simulink model "FaultCheck"  (R2022b)
settings: Solver=FixedStepAuto  StartTime=0.0  StopTime=10  FixedStep=1  RelTol=1e-3
undefined symbols (not defined in the file): C_Flt_IGBTULowerTempConfirmTh_u16, C_Flt_IGBTULowerTempDiagEn_b, C_Flt_IGBTULowerTempErrCode_u16, C_Flt_IGBTULowerTempPowerCoeff, C_Flt_IGBTULowerTempRecoveryTh_u16, C_Flt_IGBTULowerTempRecTh_s32, C_Flt_IGBTULowerTempTrigTh_s32, C_Flt_IGBTUOverTempConfirmTh_u16, C_Flt_IGBTUOverTempDiagEn_b, C_Flt_IGBTUOverTempErrCode_u16, C_Flt_IGBTUOverTempRecoveryTh_u16, C_Flt_IGBTUOverTempRecTh_s32, C_Flt_IGBTUOverTempTrigTh_s32, C_Flt_IGBTVLowerTempConfirmTh_u16, C_Flt_IGBTVLowerTempDiagEn_b, C_Flt_IGBTVLowerTempErrCode_u16, C_Flt_IGBTVLowerTempPowerCoeff, C_Flt_IGBTVLowerTempRecoveryTh_u16, C_Flt_IGBTVLowerTempRecTh_s32, C_Flt_IGBTVLowerTempTrigTh_s32, C_Flt_IGBTVOverTempConfirmTh_u16, C_Flt_IGBTVOverTempDiagEn_b, C_Flt_IGBTVOverTempErrCode_u16, C_Flt_IGBTVOverTempRecoveryTh_u16, C_Flt_IGBTVOverTempRecTh_s32, C_Flt_IGBTVOverTempTrigTh_s32, C_Flt_IGBTWLowerTempConfirmTh_u16, C_Flt_IGBTWLowerTempDiagEn_b, C_Flt_IGBTWLowerTempErrCode_u16, C_Flt_IGBTWLowerTempPowerCoeff, C_Flt_IGBTWLowerTempRecoveryTh_u16, C_Flt_IGBTWLowerTempRecTh_s32, C_Flt_IGBTWLowerTempTrigTh_s32, C_Flt_IGBTWOverTempConfirmTh_u16, C_Flt_IGBTWOverTempDiagEn_b, C_Flt_IGBTWOverTempErrCode_u16, C_Flt_IGBTWOverTempRecoveryTh_u16, C_Flt_IGBTWOverTempRecTh_s32, C_Flt_IGBTWOverTempTrigTh_s32, C_Flt_IuOCConfirmTh_u16, C_Flt_IuOCDiagEn_b, C_Flt_IuOCErrCode_u16, C_Flt_IuOCNegLimit_s32, C_Flt_IuOCPosLimit_s32, C_Flt_IuOCRecoveryTh_u16, C_Flt_IuZeroDriftDiagEn_b, C_Flt_IuZeroDriftErrCode_u16, C_Flt_IvOCConfirmTh_u16, C_Flt_IvOCDiagEn_b, C_Flt_IvOCErrCode_u16, C_Flt_IvOCNegLimit_s32, C_Flt_IvOCPosLimit_s32, C_Flt_IvOCRecoveryTh_u16, C_Flt_IvZeroDriftDiagEn_b, C_Flt_IvZeroDriftErrCode_u16, C_Flt_IwOCConfirmTh_u16, C_Flt_IwOCDiagEn_b, C_Flt_IwOCErrCode_u16, C_Flt_IwOCNegLimit_s32, C_Flt_IwOCPosLimit_s32 ... (+196)
libraries: YS_UserDefined_Library x21, simulink x5
(part 3 of 11)

== system FaultCheck/FaultDiagnose/UdcOverOneDiag/Diagnose ==
  DiagEnOut : Inport
  Udc : Inport  Port=2
  Parameter : Inport  Port=3
  Disable : Subsystem  TreatAsAtomicUnit=on
  If : If  IfExpression=u1 == 0
  Merge : Merge
  NormalDiag : Subsystem  TreatAsAtomicUnit=on
  UdcOverOneFlgOut : Outport
  wires:
  DiagEnOut/1 -> If/1
  If/1 -> Disable/Action
  If/2 -> NormalDiag/Action
  Udc/1 -> NormalDiag/1(Udc)
  Parameter/1 -> NormalDiag/2(Parameter)
  Disable/1(UdcOverOneFltDeb) -> Merge/1
  NormalDiag/1(UdcOverOneFltDeb) -> Merge/2
  Merge/1 -> UdcOverOneFlgOut/1  "M_Flt_UdcOverOneFlgOut_b"

== system FaultCheck/FaultDiagnose/UdcOverOneDiag/EnableJudgement ==
  SysSelfCheckDownFlg : Inport
  DiagEn : Inport  Port=2
  Constant : Constant  Value=true
  Logical Operator : Logic  AllPortsSameDT=off  OutDataTypeStr=boolean
  Logical Operator1 : Logic  AllPortsSameDT=off  OutDataTypeStr=boolean
  Logical Operator2 : Logic  AllPortsSameDT=off  OutDataTypeStr=boolean
  DiagEnOut : Outport
  wires:
  SysSelfCheckDownFlg/1 -> Logical Operator/2
  DiagEn/1 -> Logical Operator1/2
  Constant/1 -> Logical Operator/1, Logical Operator1/1
  Logical Operator/1 -> Logical Operator2/1
  Logical Operator1/1 -> Logical Operator2/2
  Logical Operator2/1 -> DiagEnOut/1  "M_Flt_UdcOverOneDiagEn_b"

== system FaultCheck/FaultDiagnose/UdcOverOneDiag/FaultLevelDeter ==
  UdcOverOneFlgOut : Inport
  FaultLevel : Inport  Port=2
  If : If  IfExpression=u1 == 0
  Merge : Merge
  Normal : Subsystem  TreatAsAtomicUnit=on
  OverOne : Subsystem  TreatAsAtomicUnit=on
  UdcOverOneFltLevelOut : Outport
  wires:
  UdcOverOneFlgOut/1 -> If/1
  If/1 -> Normal/Action
  If/2 -> OverOne/Action
  Normal/1(UdcOverOneFltLevel) -> Merge/1
  OverOne/1(UdcOverOneFltLevel) -> Merge/2
  Merge/1 -> UdcOverOneFltLevelOut/1  "M_Flt_UdcOverOneFltLevelOut_u8"
  FaultLevel/1 -> OverOne/1(FaultLevel)

== system FaultCheck/FaultDiagnose/UdcOverOneDiag/Parameter ==
  Udc : Inport
  1-D Lookup Table : Lookup_n-D  NumberOfTableDimensions=1  BreakpointsForDimension1=[-5:5]  BreakpointsForDimension1DataTypeStr=Inherit: Inherit from 'Breakpoint data'  IndexSearchMethod=Linear search  Table=tanh([-5:5])  TableDataTypeStr=Inherit: Inherit from 'Table data'  ExtrapMethod=Clip  UseLastTableValue=on  InternalRulePriority=Speed  OutDataTypeStr=single  RndMeth=Simplest
  Bus Creator : BusCreator  Inputs=8
  Constant : Constant  Value=C_Flt_UdcOverOneDiagEn_b
  Constant1 : Constant  Value=C_Flt_UdcOverOneErrCode_u16
  Constant2 : Constant  Value=C_Flt_UdcOverOneConfirmTh_u16
  Constant3 : Constant  Value=C_Flt_UdcOverOneRecoveryTh_u16
  Constant4 : Constant  Value=C_Flt_UdcOverOneTrigTh_s32
  Constant5 : Constant  Value=C_Flt_UdcOverOneRecTh_s32
  Constant6 : Constant  Value=C_Flt_LevelTwo_u8
  Parameter : Outport
  wires:
  Bus Creator/1 -> Parameter/1
  Constant/1 -> Bus Creator/1  "UdcOverOneDiagEn"
  Udc/1 -> 1-D Lookup Table/1
  Constant1/1 -> Bus Creator/2  "UdcOverOneErrCode"
  Constant2/1 -> Bus Creator/5  "UdcOverOneConfirmTh"
  Constant3/1 -> Bus Creator/6  "UdcOverOneRecoveryTh"
  Constant6/1 -> Bus Creator/7  "UdcOverOneFltLevel"
  1-D Lookup Table/1 -> Bus Creator/8  "UdcOverOnePowerCoeff"
  Constant4/1 -> Bus Creator/3  "UdcOverOneTrigTh"
  Constant5/1 -> Bus Creator/4  "UdcOverOneRecTh"

== system FaultCheck/FaultDiagnose/UdcOverOneDiag/PowerReductionCoeffDeter ==
  UdcOverOneFltLevelOut : Inport
  PowerCoeff : Inport  Port=2
  If : If  IfExpression=u1 < 2  ElseIfExpressions=u1 == 2
  If Action Subsystem : Subsystem  TreatAsAtomicUnit=on
  If Action Subsystem1 : Subsystem  TreatAsAtomicUnit=on
  If Action Subsystem2 : Subsystem  TreatAsAtomicUnit=on
  Merge : Merge  Inputs=3
  UdcOverOnePowerCoeffOut : Outport
  wires:
  UdcOverOneFltLevelOut/1 -> If/1
  If/1 -> If Action Subsystem/Action
  If/2 -> If Action Subsystem1/Action
  If/3 -> If Action Subsystem2/Action
  PowerCoeff/1 -> If Action Subsystem1/1(PowerCoeff)
  If Action Subsystem/1(Coeff) -> Merge/1
  If Action Subsystem1/1(Coeff) -> Merge/2
  If Action Subsystem2/1(Coeff) -> Merge/3
  Merge/1 -> UdcOverOnePowerCoeffOut/1  "M_Flt_UdcOverOnePowerCoeffOut_s32"

== system FaultCheck/FaultDiagnose/UdcOverTwoDiag/Diagnose ==
  DiagEnOut : Inport
  Udc : Inport  Port=2
  Parameter : Inport  Port=3
  Disable : Subsystem  TreatAsAtomicUnit=on
  If : If  IfExpression=u1 == 0
  Merge : Merge
  NormalDiag : Subsystem  TreatAsAtomicUnit=on
  UdcOverTwoFlgOut : Outport
  wires:
  DiagEnOut/1 -> If/1
  If/1 -> Disable/Action
  If/2 -> NormalDiag/Action
  Udc/1 -> NormalDiag/1(Udc)
  Parameter/1 -> NormalDiag/2(Parameter)
  Disable/1(UdcOverTwoFltDeb) -> Merge/1
  NormalDiag/1(UdcOverTwoFltDeb) -> Merge/2
  Merge/1 -> UdcOverTwoFlgOut/1  "M_Flt_UdcOverTwoFlgOut_b"

== system FaultCheck/FaultDiagnose/UdcOverTwoDiag/EnableJudgement ==
  SysSelfCheckDownFlg : Inport
  DiagEn : Inport  Port=2
  Constant : Constant  Value=true
  Logical Operator : Logic  AllPortsSameDT=off  OutDataTypeStr=boolean
  Logical Operator1 : Logic  AllPortsSameDT=off  OutDataTypeStr=boolean
  Logical Operator2 : Logic  AllPortsSameDT=off  OutDataTypeStr=boolean
  DiagEnOut : Outport
  wires:
  SysSelfCheckDownFlg/1 -> Logical Operator/2
  DiagEn/1 -> Logical Operator1/2
  Constant/1 -> Logical Operator/1, Logical Operator1/1
  Logical Operator/1 -> Logical Operator2/1
  Logical Operator1/1 -> Logical Operator2/2
  Logical Operator2/1 -> DiagEnOut/1  "M_Flt_UdcOverTwoDiagEn_b"

== system FaultCheck/FaultDiagnose/UdcOverTwoDiag/FaultLevelDeter ==
  UdcOverTwoFlgOut : Inport
  FaultLevel : Inport  Port=2
  If : If  IfExpression=u1 == 0
  Merge : Merge
  Normal : Subsystem  TreatAsAtomicUnit=on
  OverTwo : Subsystem  TreatAsAtomicUnit=on
  UdcOverTwoFltLevelOut : Outport
  wires:
  UdcOverTwoFlgOut/1 -> If/1
  If/1 -> Normal/Action
  If/2 -> OverTwo/Action
  Normal/1(UdcOverTwoFltLevel) -> Merge/1
  OverTwo/1(UdcOverTwoFltLevel) -> Merge/2
  Merge/1 -> UdcOverTwoFltLevelOut/1  "M_Flt_UdcOverTwoFltLevelOut_u8"
  FaultLevel/1 -> OverTwo/1(FaultLevel)

== system FaultCheck/FaultDiagnose/UdcOverTwoDiag/Parameter ==
  Bus Creator : BusCreator  Inputs=7
  Constant : Constant  Value=C_Flt_UdcOverTwoDiagEn_b
  Constant1 : Constant  Value=C_Flt_UdcOverTwoErrCode_u16
  Constant2 : Constant  Value=C_Flt_UdcOverTwoConfirmTh_u16
  Constant3 : Constant  Value=C_Flt_UdcOverTwoRecoveryTh_u16
  Constant4 : Constant  Value=C_Flt_UdcOverTwoTrigTh_s32
  Constant5 : Constant  Value=C_Flt_PowerCoeffZero_s32
  Constant6 : Constant  Value=C_Flt_LevelFive_u8
  Parameter : Outport
  wires:
  Bus Creator/1 -> Parameter/1
  Constant/1 -> Bus Creator/1  "UdcOverTwoDiagEn"
  Constant1/1 -> Bus Creator/2  "UdcOverTwoErrCode"
  Constant2/1 -> Bus Creator/4  "UdcOverTwoConfirmTh"
  Constant3/1 -> Bus Creator/5  "UdcOverTwoRecoveryTh"
  Constant6/1 -> Bus Creator/6  "UdcOverTwoFltLevel"
  Constant5/1 -> Bus Creator/7  "UdcOverTwoPowerCoeff"
  Constant4/1 -> Bus Creator/3  "UdcOverTwoTrigTh"

== system FaultCheck/FaultDiagnose/UdcOverTwoDiag/PowerReductionCoeffDeter ==
  UdcOverTwoFltLevelOut : Inport
  PowerCoeff : Inport  Port=2
  If : If  IfExpression=u1 < 2  ElseIfExpressions=u1 == 2
  If Action Subsystem : Subsystem  TreatAsAtomicUnit=on
  If Action Subsystem1 : Subsystem  TreatAsAtomicUnit=on
  If Action Subsystem2 : Subsystem  TreatAsAtomicUnit=on
  Merge : Merge  Inputs=3
  UdcOverTwoPowerCoeffOut : Outport
  wires:
  UdcOverTwoFltLevelOut/1 -> If/1
  If/1 -> If Action Subsystem/Action
  If/2 -> If Action Subsystem1/Action
  If/3 -> If Action Subsystem2/Action
  PowerCoeff/1 -> If Action Subsystem1/1(PowerCoeff)
  If Action Subsystem/1(Coeff) -> Merge/1
  If Action Subsystem1/1(Coeff) -> Merge/2
  If Action Subsystem2/1(Coeff) -> Merge/3
  Merge/1 -> UdcOverTwoPowerCoeffOut/1  "M_Flt_UdcOverTwoPowerCoeffOut_s32"

== system FaultCheck/FltCheck/Determination/Detection Criteria ==
  FltSrc : Inport
  FltTh : Inport  Port=2
  Condition : Inport  Port=3
  Determination : Subsystem
  Equal : Subsystem
  Lower : Subsystem
  NotEqual : Subsystem
  Overflow : Subsystem
  Fail : Outport
  wires:
  FltTh/1 -> NotEqual/2(FltTh), Lower/2(FltTh), Overflow/2(FltTh), Equal/2(FltTh)
  FltSrc/1 -> NotEqual/1(FltSrc), Lower/1(FltSrc), Overflow/1(FltSrc), Equal/1(FltSrc)
  Equal/1(EQ) -> Determination/2(EQ)
  Overflow/1(GT) -> Determination/3(GT)
  Lower/1(LT) -> Determination/4(LT)
  NotEqual/1(NEQ) -> Determination/5(NEQ)
  Condition/1 -> Determination/1(Condition)
  Determination/1(Fail) -> Fail/1

== system FaultCheck/FltCheck/Determination/Hysteresis ==
  Fail : Inport
  ConfirmTh : Inport  Port=2
  ClearTh : Inport  Port=3
  FastRecover_one : Inport  Port=4
  Hysteresis_Chart : Stateflow chart  TreatAsAtomicUnit=on
  Out : Outport
  wires:
  Fail/1 -> Hysteresis_Chart/1(Fail)
  ClearTh/1 -> Hysteresis_Chart/2(ClearTh)
  ConfirmTh/1 -> Hysteresis_Chart/3(ConfirmTh)
  FastRecover_one/1 -> Hysteresis_Chart/4(FastRecover_one)
  Hysteresis_Chart/1(Out) -> Out/1

== system FaultCheck/FaultDiag_HighTask_100us/FltDetn/CurrentSensorDetn/Enable ==
  Sys_SelfChkFishFlg : Inport
  Constant : Constant  Value=FLT_ON
  Constant1 : Constant  Value=FLT_ON
  Constant2 : Constant  Value=FLT_OFF
  Relational Operator : RelationalOperator  Operator===  OutDataTypeStr=boolean  RndMeth=Simplest  InputSameDT=off
  Switch : Switch  Criteria=u2 > Threshold  SaturateOnIntegerOverflow=off  InputSameDT=off
  Enable : Outport
  wires:
  Switch/1 -> Enable/1
  Constant2/1 -> Switch/3
  Constant1/1 -> Switch/1
  Relational Operator/1 -> Switch/2
  Constant/1 -> Relational Operator/2
  Sys_SelfChkFishFlg/1 -> Relational Operator/1

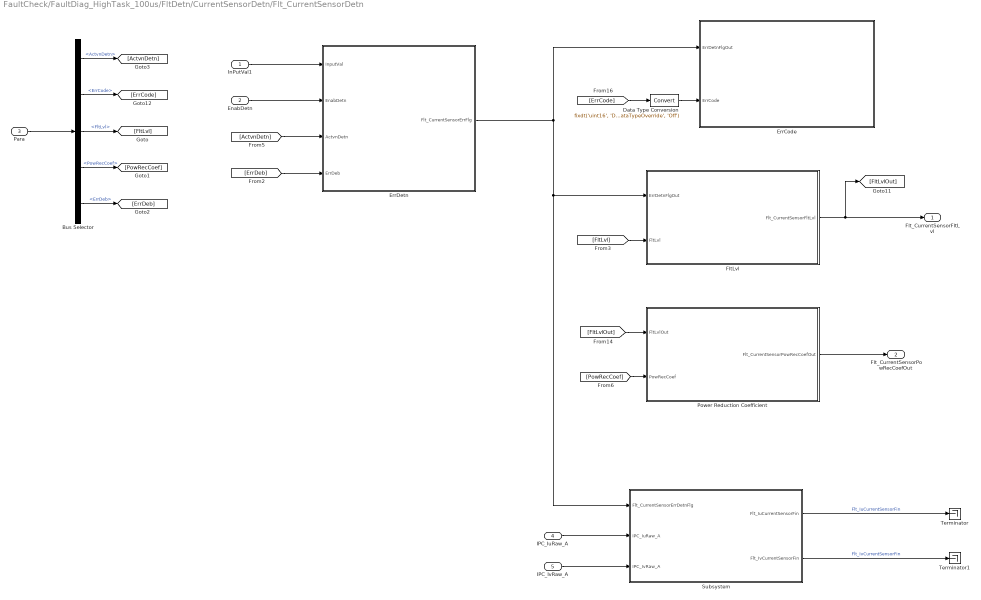
== system FaultCheck/FaultDiag_HighTask_100us/FltDetn/CurrentSensorDetn/Flt_CurrentSensorDetn ==
  InPutVal1 : Inport
  EnabDetn : Inport  Port=2
  Para : Inport  Port=3
  IPC_IuRaw_A : Inport  Port=4
  IPC_IvRaw_A : Inport  Port=5
  Bus Selector : BusSelector  OutputSignals=ActvnDetn,ErrCode,FltLvl,PowRecCoef,ErrDeb
  Data Type Conversion : DataTypeConversion  OutDataTypeStr=fixdt('uint16', 'DataTypeOverride', 'Off')  SaturateOnIntegerOverflow=off  RndMeth=Floor
  ErrCode : Subsystem
  ErrDetn : Subsystem
  FltLvl : Subsystem
  Power Reduction Coefficient : Subsystem
  Subsystem : Subsystem
  Terminator : Terminator
  Terminator1 : Terminator
  Flt_CurrentSensorFltLvl : Outport
  Flt_CurrentSensorPowRecCoefOut : Outport  Port=2
  wires:
  Subsystem/2(Flt_IvCurrentSensorFin) -> Terminator1/1  "Flt_IvCurrentSensorFin"
  IPC_IvRaw_A/1 -> Subsystem/3(IPC_IvRaw_A)
  IPC_IuRaw_A/1 -> Subsystem/2(IPC_IuRaw_A)
  Subsystem/1(Flt_IuCurrentSensorFin) -> Terminator/1  "Flt_IuCurrentSensorFin"
  ErrDetn/1(Flt_CurrentSensorErrFlg) -> Subsystem/1(Flt_CurrentSensorErrDetnFlg), FltLvl/1(ErrDetnFlgOut), ErrCode/1(ErrDetnFlgOut)
  Bus Selector/5 -> [ErrDeb]  "<ErrDeb>"
  InPutVal1/1 -> ErrDetn/1(InputVal)
  [ActvnDetn] -> ErrDetn/3(ActvnDetn)
  EnabDetn/1 -> ErrDetn/2(EnabDetn)
  [ErrDeb] -> ErrDetn/4(ErrDeb)
  Bus Selector/4 -> [PowRecCoef]  "<PowRecCoef>"
  Bus Selector/3 -> [FltLvl]  "<FltLvl>"
  Bus Selector/2 -> [ErrCode]  "<ErrCode>"
  Bus Selector/1 -> [ActvnDetn]  "<ActvnDetn>"
  Para/1 -> Bus Selector/1
  [ErrCode] -> Data Type Conversion/1
  FltLvl/1(Flt_CurrentSensorFltLvl) -> [FltLvlOut], Flt_CurrentSensorFltLvl/1
  [FltLvl] -> FltLvl/2(FltLvl)
  [FltLvlOut] -> Power Reduction Coefficient/1(FltLvlOut)
  [PowRecCoef] -> Power Reduction Coefficient/2(PowRecCoef)
  Power Reduction Coefficient/1(Flt_CurrentSensorPowRecCoefOut) -> Flt_CurrentSensorPowRecCoefOut/1
  Data Type Conversion/1 -> ErrCode/2(ErrCode)

== system FaultCheck/FaultDiag_HighTask_100us/FltDetn/CurrentSensorDetn/Parameter ==
  Bus Creator : BusCreator  Inputs=5
  Constant2 : Constant  Value=FLT_COEF_ZERO
  Constant3 : Constant  Value=Flt_CurrentSensor_ErrCode
  Constant4 : Constant  Value=FLTLVL_FOUR
  Constant5 : Constant  Value=Flt_CurrentSensor_ActvnDetn
  Constant8 : Constant  Value=Flt_CurrentSensor_ErrDeb
  Para : Outport
  wires:
  Constant8/1 -> Bus Creator/1  "ErrDeb"
  Constant2/1 -> Bus Creator/5  "PowRecCoef"
  Constant3/1 -> Bus Creator/3  "ErrCode"
  Constant5/1 -> Bus Creator/2  "ActvnDetn"
  Constant4/1 -> Bus Creator/4  "FltLvl"
  Bus Creator/1 -> Para/1

== system FaultCheck/FaultDiag_HighTask_100us/FltDetn/CurrentZeroDrfDetn/CurrZeroDrfDetn ==
  InPutVal : Inport
  EnabDetn : Inport  Port=2
  Para : Inport  Port=3
  Bus Selector : BusSelector  OutputSignals=ActvnDetn,ErrCode,FltLvl,PowRecCoef
  ErrCode1 : Subsystem
  ErrDetn : Subsystem
  FltLvl : Subsystem
  Power Reduction Coefficient : Subsystem
  Flt_CurrZeroDrfFltLvl : Outport
  Flt_CurrZeroDrfPowRecCoefOut : Outport  Port=2
  wires:
  ErrDetn/1(Flt_CurrZeroDrfErrFlg) -> FltLvl/1(ErrDetnFlgOut), ErrCode1/1(ErrDetnFlgOut)
  InPutVal/1 -> ErrDetn/1(InputVal)
  [ActvnDetn] -> ErrDetn/3(ActvnDetn)
  EnabDetn/1 -> ErrDetn/2(EnabDetn)
  Bus Selector/4 -> [PowRecCoef]  "<PowRecCoef>"
  Bus Selector/3 -> [FltLvl]  "<FltLvl>"
  Bus Selector/2 -> [ErrCode]  "<ErrCode>"
  Bus Selector/1 -> [ActvnDetn]  "<ActvnDetn>"
  Para/1 -> Bus Selector/1
  [ErrCode] -> ErrCode1/2(ErrCode)
  FltLvl/1(Flt_CurrZeroDrfFltLvl) -> [FltLvlOut], Flt_CurrZeroDrfFltLvl/1
  [FltLvl] -> FltLvl/2(FltLvl)
  [FltLvlOut] -> Power Reduction Coefficient/1(FltLvlOut)
  [PowRecCoef] -> Power Reduction Coefficient/2(PowRecCoef)
  Power Reduction Coefficient/1(Flt_CurrZeroDrfPowRecCoefOut) -> Flt_CurrZeroDrfPowRecCoefOut/1

== system FaultCheck/FaultDiag_HighTask_100us/FltDetn/CurrentZeroDrfDetn/Enable ==
  Constant : Constant  Value=FLT_ON
  Enable : Outport
  wires:
  Constant/1 -> Enable/1

== system FaultCheck/FaultDiag_HighTask_100us/FltDetn/CurrentZeroDrfDetn/Parameter ==
  Bus Creator : BusCreator  Inputs=4
  Constant2 : Constant  Value=FLT_COEF_ZERO
  Constant3 : Constant  Value=Flt_CurrZeroDrf_ErrCode
  Constant4 : Constant  Value=FLTLVL_FIVE
  Constant5 : Constant  Value=Flt_CurrZeroDrf_ActvnErrDetn
  Para : Outport
  wires:
  Constant2/1 -> Bus Creator/4  "PowRecCoef"
  Constant3/1 -> Bus Creator/2  "ErrCode"
  Constant5/1 -> Bus Creator/1  "ActvnDetn"
  Constant4/1 -> Bus Creator/3  "FltLvl"
  Bus Creator/1 -> Para/1

== system FaultCheck/FaultDiag_HighTask_100us/FltDetn/DriveUdcDetn/DriveUdcDetn ==
  InPutVal1 : Inport
  EnabDetn : Inport  Port=2
  Para : Inport  Port=3
  Bus Selector : BusSelector  OutputSignals=ActvnDetn,ErrCode,FltLvl,PowRecCoef,ErrDeb
  ErrCode : Subsystem
  ErrDetn : Subsystem
  FltLvl : Subsystem
  Power Reduction Coefficient : Subsystem
  Flt_DriveUdcFltLvl : Outport
  Flt_DriveUdcPowRecCoefOut : Outport  Port=2
  wires:
  Power Reduction Coefficient/1(Flt_DriveUdcPowRecCoefOut) -> Flt_DriveUdcPowRecCoefOut/1
  [PowRecCoef] -> Power Reduction Coefficient/2(PowRecCoef)
  [FltLvlOut] -> Power Reduction Coefficient/1(FltLvlOut)
  [FltLvl] -> FltLvl/2(FltLvl)
  FltLvl/1(Flt_DriveUdcFltLvl) -> Flt_DriveUdcFltLvl/1, [FltLvlOut]
  [ErrCode] -> ErrCode/2(ErrCode)
  Para/1 -> Bus Selector/1
  Bus Selector/1 -> [ActvnDetn]  "<ActvnDetn>"
  Bus Selector/2 -> [ErrCode]  "<ErrCode>"
  Bus Selector/3 -> [FltLvl]  "<FltLvl>"
  Bus Selector/4 -> [PowRecCoef]  "<PowRecCoef>"
  [ErrDeb] -> ErrDetn/4(ErrDeb)
  EnabDetn/1 -> ErrDetn/2(EnabDetn)
  [ActvnDetn] -> ErrDetn/3(ActvnDetn)
  InPutVal1/1 -> ErrDetn/1(InputVal)
  ErrDetn/1(Flt_DriveUdcErrFlg) -> ErrCode/1(ErrDetnFlgOut), FltLvl/1(ErrDetnFlgOut)
  Bus Selector/5 -> [ErrDeb]  "<ErrDeb>"

== system FaultCheck/FaultDiag_HighTask_100us/FltDetn/DriveUdcDetn/Enable ==
  Sys_SelfChkFishFlg : Inport
  Constant : Constant  Value=FLT_ON
  Constant1 : Constant  Value=FLT_ON
  Constant2 : Constant  Value=FLT_OFF
  Relational Operator : RelationalOperator  Operator===  OutDataTypeStr=boolean  RndMeth=Simplest  InputSameDT=off
  Switch : Switch  Criteria=u2 > Threshold  SaturateOnIntegerOverflow=off  InputSameDT=off
  Enable : Outport
  wires:
  Sys_SelfChkFishFlg/1 -> Relational Operator/1
  Constant/1 -> Relational Operator/2
  Relational Operator/1 -> Switch/2
  Constant1/1 -> Switch/1
  Constant2/1 -> Switch/3
  Switch/1 -> Enable/1

== system FaultCheck/FaultDiag_HighTask_100us/FltDetn/DriveUdcDetn/Parameter ==
  Bus Creator : BusCreator  Inputs=5
  Constant2 : Constant  Value=FLT_COEF_ZERO
  Constant3 : Constant  Value=Flt_DriveUdc_ErrCode
  Constant4 : Constant  Value=FLTLVL_FOUR
  Constant5 : Constant  Value=Flt_DriveUdc_ActvnDetn
  Constant8 : Constant  Value=Flt_DriveUdc_ErrDeb
  Para : Outport
  wires:
  Bus Creator/1 -> Para/1
  Constant4/1 -> Bus Creator/4  "FltLvl"
  Constant5/1 -> Bus Creator/2  "ActvnDetn"
  Constant3/1 -> Bus Creator/3  "ErrCode"
  Constant2/1 -> Bus Creator/5  "PowRecCoef"
  Constant8/1 -> Bus Creator/1  "ErrDeb"

== system FaultCheck/FaultDiag_HighTask_100us/FltDetn/Drive_H_Detn/Drive_H_Detn ==
  InPutVal1 : Inport
  EnabDetn : Inport  Port=2
  Para : Inport  Port=3
  Bus Selector : BusSelector  OutputSignals=ActvnDetn,ErrCode,FltLvl,PowRecCoef,ErrDeb
  ErrCode : Subsystem
  ErrDetn : Subsystem
  FltLvl : Subsystem
  Power Reduction Coefficient : Subsystem
  Flt_Drive_H_FltLvl : Outport
  Flt_Drive_H_PowRecCoefOut : Outport  Port=2
  wires:
  Power Reduction Coefficient/1(Flt_Drive_H_PowRecCoefOut) -> Flt_Drive_H_PowRecCoefOut/1
  [PowRecCoef] -> Power Reduction Coefficient/2(PowRecCoef)
  [FltLvlOut] -> Power Reduction Coefficient/1(FltLvlOut)
  [FltLvl] -> FltLvl/2(FltLvl)
  FltLvl/1(Flt_Drive_H_FltLvl) -> Flt_Drive_H_FltLvl/1, [FltLvlOut]
  [ErrCode] -> ErrCode/2(ErrCode)
  Para/1 -> Bus Selector/1
  Bus Selector/1 -> [ActvnDetn]  "<ActvnDetn>"
  Bus Selector/2 -> [ErrCode]  "<ErrCode>"
  Bus Selector/3 -> [FltLvl]  "<FltLvl>"
  Bus Selector/4 -> [PowRecCoef]  "<PowRecCoef>"
  [ErrDeb] -> ErrDetn/4(ErrDeb)
  EnabDetn/1 -> ErrDetn/2(EnabDetn)
  [ActvnDetn] -> ErrDetn/3(ActvnDetn)
  InPutVal1/1 -> ErrDetn/1(InputVal)
  ErrDetn/1(Flt_Drive_H_ErrFlg) -> ErrCode/1(ErrDetnFlgOut), FltLvl/1(ErrDetnFlgOut)
  Bus Selector/5 -> [ErrDeb]  "<ErrDeb>"

== system FaultCheck/FaultDiag_HighTask_100us/FltDetn/Drive_H_Detn/Enable ==
  Sys_SelfChkFishFlg : Inport
  Constant : Constant  Value=FLT_ON
  Constant1 : Constant  Value=FLT_ON
  Constant2 : Constant  Value=FLT_OFF
  Relational Operator : RelationalOperator  Operator===  OutDataTypeStr=boolean  RndMeth=Simplest  InputSameDT=off
  Switch : Switch  Criteria=u2 > Threshold  SaturateOnIntegerOverflow=off  InputSameDT=off
  Enable : Outport
  wires:
  Sys_SelfChkFishFlg/1 -> Relational Operator/1
  Constant/1 -> Relational Operator/2
  Relational Operator/1 -> Switch/2
  Constant1/1 -> Switch/1
  Constant2/1 -> Switch/3
  Switch/1 -> Enable/1

== system FaultCheck/FaultDiag_HighTask_100us/FltDetn/Drive_H_Detn/Parameter ==
  Bus Creator : BusCreator  Inputs=5
  Constant2 : Constant  Value=FLT_COEF_ZERO
  Constant3 : Constant  Value=Flt_Drive_H_ErrCode
  Constant4 : Constant  Value=FLTLVL_FOUR
  Constant5 : Constant  Value=Flt_Drive_H_ActvnDetn
  Constant8 : Constant  Value=Flt_Drive_H_ErrDeb
  Para : Outport
  wires:
  Bus Creator/1 -> Para/1
  Constant4/1 -> Bus Creator/4  "FltLvl"
  Constant5/1 -> Bus Creator/2  "ActvnDetn"
  Constant3/1 -> Bus Creator/3  "ErrCode"
  Constant2/1 -> Bus Creator/5  "PowRecCoef"
  Constant8/1 -> Bus Creator/1  "ErrDeb"

== system FaultCheck/FaultDiag_HighTask_100us/FltDetn/Drive_L_Detn/Drive_L_Detn ==
  InPutVal1 : Inport
  EnabDetn : Inport  Port=2
  Para : Inport  Port=3
  Bus Selector : BusSelector  OutputSignals=ActvnDetn,ErrCode,FltLvl,PowRecCoef,ErrDeb
  ErrCode : Subsystem
  ErrDetn : Subsystem
  FltLvl : Subsystem
  Power Reduction Coefficient : Subsystem
  Flt_Drive_L_FltLvl : Outport
  Flt_Drive_L_PowRecCoefOut : Outport  Port=2
  wires:
  Power Reduction Coefficient/1(Flt_Drive_L_PowRecCoefOut) -> Flt_Drive_L_PowRecCoefOut/1
  [PowRecCoef] -> Power Reduction Coefficient/2(PowRecCoef)
  [FltLvlOut] -> Power Reduction Coefficient/1(FltLvlOut)
  [FltLvl] -> FltLvl/2(FltLvl)
  FltLvl/1(Flt_Drive_L_FltLvl) -> Flt_Drive_L_FltLvl/1, [FltLvlOut]
  [ErrCode] -> ErrCode/2(ErrCode)
  Para/1 -> Bus Selector/1
  Bus Selector/1 -> [ActvnDetn]  "<ActvnDetn>"
  Bus Selector/2 -> [ErrCode]  "<ErrCode>"
  Bus Selector/3 -> [FltLvl]  "<FltLvl>"
  Bus Selector/4 -> [PowRecCoef]  "<PowRecCoef>"
  [ErrDeb] -> ErrDetn/4(ErrDeb)
  EnabDetn/1 -> ErrDetn/2(EnabDetn)
  [ActvnDetn] -> ErrDetn/3(ActvnDetn)
  InPutVal1/1 -> ErrDetn/1(InputVal)
  ErrDetn/1(Flt_Drive_L_ErrFlg) -> ErrCode/1(ErrDetnFlgOut), FltLvl/1(ErrDetnFlgOut)
  Bus Selector/5 -> [ErrDeb]  "<ErrDeb>"

== system FaultCheck/FaultDiag_HighTask_100us/FltDetn/Drive_L_Detn/Enable ==
  Sys_SelfChkFishFlg : Inport
  Constant : Constant  Value=FLT_ON
  Constant1 : Constant  Value=FLT_ON
  Constant2 : Constant  Value=FLT_OFF
  Relational Operator : RelationalOperator  Operator===  OutDataTypeStr=boolean  RndMeth=Simplest  InputSameDT=off
  Switch : Switch  Criteria=u2 > Threshold  SaturateOnIntegerOverflow=off  InputSameDT=off
  Enable : Outport
  wires:
  Sys_SelfChkFishFlg/1 -> Relational Operator/1
  Constant/1 -> Relational Operator/2
  Relational Operator/1 -> Switch/2
  Constant1/1 -> Switch/1
  Constant2/1 -> Switch/3
  Switch/1 -> Enable/1

== system FaultCheck/FaultDiag_HighTask_100us/FltDetn/Drive_L_Detn/Parameter ==
  Bus Creator : BusCreator  Inputs=5
  Constant2 : Constant  Value=FLT_COEF_ZERO
  Constant3 : Constant  Value=Flt_Drive_L_ErrCode
  Constant4 : Constant  Value=FLTLVL_FOUR
  Constant5 : Constant  Value=Flt_Drive_L_ActvnDetn
  Constant8 : Constant  Value=Flt_Drive_L_ErrDeb
  Para : Outport
  wires:
  Bus Creator/1 -> Para/1
  Constant4/1 -> Bus Creator/4  "FltLvl"
  Constant5/1 -> Bus Creator/2  "ActvnDetn"
  Constant3/1 -> Bus Creator/3  "ErrCode"
  Constant2/1 -> Bus Creator/5  "PowRecCoef"
  Constant8/1 -> Bus Creator/1  "ErrDeb"

== system FaultCheck/FaultDiag_HighTask_100us/FltDetn/HWOverCurrDetn/Enable ==
  Sys_SelfChkFishFlg : Inport
  Constant : Constant  Value=FLT_ON
  Constant1 : Constant  Value=FLT_ON
  Constant2 : Constant  Value=FLT_OFF
  Relational Operator : RelationalOperator  Operator===  OutDataTypeStr=boolean  RndMeth=Simplest  InputSameDT=off
  Switch : Switch  Criteria=u2 > Threshold  SaturateOnIntegerOverflow=off  InputSameDT=off
  Enable : Outport
  wires:
  Sys_SelfChkFishFlg/1 -> Relational Operator/1
  Constant/1 -> Relational Operator/2
  Relational Operator/1 -> Switch/2
  Constant1/1 -> Switch/1
  Constant2/1 -> Switch/3
  Switch/1 -> Enable/1

== system FaultCheck/FaultDiag_HighTask_100us/FltDetn/HWOverCurrDetn/HWOverCurrDetn ==
  InPutVal1 : Inport
  EnabDetn : Inport  Port=2
  Para : Inport  Port=3
  Bus Selector : BusSelector  OutputSignals=ActvnDetn,ErrCode,FltLvl,PowRecCoef,ErrDeb
  ErrCode : Subsystem
  ErrDetn : Subsystem
  FltLvl : Subsystem
  Power Reduction Coefficient : Subsystem
  Flt_HWOverCurrFltLvl : Outport
  Flt_HWOverCurrPowRecCoefOut : Outport  Port=2
  wires:
  Power Reduction Coefficient/1(Flt_HWOverCurrPowRecCoefOut) -> Flt_HWOverCurrPowRecCoefOut/1
  [PowRecCoef] -> Power Reduction Coefficient/2(PowRecCoef)
  [FltLvlOut] -> Power Reduction Coefficient/1(FltLvlOut)
  [FltLvl] -> FltLvl/2(FltLvl)
  FltLvl/1(Flt_HWOverCurrFltLvl) -> Flt_HWOverCurrFltLvl/1, [FltLvlOut]
  [ErrCode] -> ErrCode/2(ErrCode)
  Para/1 -> Bus Selector/1
  Bus Selector/1 -> [ActvnDetn]  "<ActvnDetn>"
  Bus Selector/2 -> [ErrCode]  "<ErrCode>"
  Bus Selector/3 -> [FltLvl]  "<FltLvl>"
  Bus Selector/4 -> [PowRecCoef]  "<PowRecCoef>"
  [ErrDeb] -> ErrDetn/4(ErrDeb)
  EnabDetn/1 -> ErrDetn/2(EnabDetn)
  [ActvnDetn] -> ErrDetn/3(ActvnDetn)
  InPutVal1/1 -> ErrDetn/1(InputVal)
  ErrDetn/1(Flt_HWOverCurrErrFlg) -> ErrCode/1(ErrDetnFlgOut), FltLvl/1(ErrDetnFlgOut)
  Bus Selector/5 -> [ErrDeb]  "<ErrDeb>"

== system FaultCheck/FaultDiag_HighTask_100us/FltDetn/HWOverCurrDetn/Parameter ==
  Bus Creator : BusCreator  Inputs=5
  Constant2 : Constant  Value=FLT_COEF_ZERO
  Constant3 : Constant  Value=Flt_HWOverCurr_ErrCode
  Constant4 : Constant  Value=FLTLVL_FOUR
  Constant5 : Constant  Value=Flt_HWOverCurr_ActvnDetn
  Constant8 : Constant  Value=Flt_HWOverCurr_ErrDeb
  Para : Outport
  wires:
  Bus Creator/1 -> Para/1
  Constant4/1 -> Bus Creator/4  "FltLvl"
  Constant5/1 -> Bus Creator/2  "ActvnDetn"
  Constant3/1 -> Bus Creator/3  "ErrCode"
  Constant2/1 -> Bus Creator/5  "PowRecCoef"
  Constant8/1 -> Bus Creator/1  "ErrDeb"

== system FaultCheck/FaultDiag_HighTask_100us/FltDetn/HWOverUdcDetn/Enable ==
  Sys_SelfChkFishFlg : Inport
  Constant : Constant  Value=FLT_ON
  Constant1 : Constant  Value=FLT_ON
  Constant2 : Constant  Value=FLT_OFF
  Relational Operator : RelationalOperator  Operator===  OutDataTypeStr=boolean  RndMeth=Simplest  InputSameDT=off
  Switch : Switch  Criteria=u2 > Threshold  SaturateOnIntegerOverflow=off  InputSameDT=off
  Enable : Outport
  wires:
  Sys_SelfChkFishFlg/1 -> Relational Operator/1
  Constant/1 -> Relational Operator/2
  Relational Operator/1 -> Switch/2
  Constant1/1 -> Switch/1
  Constant2/1 -> Switch/3
  Switch/1 -> Enable/1

== system FaultCheck/FaultDiag_HighTask_100us/FltDetn/HWOverUdcDetn/HWOverCurrDetn ==
  InPutVal1 : Inport
  EnabDetn : Inport  Port=2
  Para : Inport  Port=3
  Bus Selector : BusSelector  OutputSignals=ActvnDetn,ErrCode,FltLvl,PowRecCoef,ErrDeb
  ErrCode : Subsystem
  ErrDetn : Subsystem
  FltLvl : Subsystem
  Power Reduction Coefficient : Subsystem
  Flt_HWOverUdcFltLvl : Outport
  Flt_HWOverUdcPowRecCoefOut : Outport  Port=2
  wires:
  Power Reduction Coefficient/1(Flt_HWOverUdcPowRecCoefOut) -> Flt_HWOverUdcPowRecCoefOut/1
  [PowRecCoef] -> Power Reduction Coefficient/2(PowRecCoef)
  [FltLvlOut] -> Power Reduction Coefficient/1(FltLvlOut)
  [FltLvl] -> FltLvl/2(FltLvl)
  FltLvl/1(Flt_HWOverUdcFltLvl) -> Flt_HWOverUdcFltLvl/1, [FltLvlOut]
  [ErrCode] -> ErrCode/2(ErrCode)
  Para/1 -> Bus Selector/1
  Bus Selector/1 -> [ActvnDetn]  "<ActvnDetn>"
  Bus Selector/2 -> [ErrCode]  "<ErrCode>"
  Bus Selector/3 -> [FltLvl]  "<FltLvl>"
  Bus Selector/4 -> [PowRecCoef]  "<PowRecCoef>"
  [ErrDeb] -> ErrDetn/4(ErrDeb)
  EnabDetn/1 -> ErrDetn/2(EnabDetn)
  [ActvnDetn] -> ErrDetn/3(ActvnDetn)
  InPutVal1/1 -> ErrDetn/1(InputVal)
  ErrDetn/1(Flt_HWOverUdcErrFlg) -> ErrCode/1(ErrDetnFlgOut), FltLvl/1(ErrDetnFlgOut)
  Bus Selector/5 -> [ErrDeb]  "<ErrDeb>"

== system FaultCheck/FaultDiag_HighTask_100us/FltDetn/HWOverUdcDetn/Parameter ==
  Bus Creator : BusCreator  Inputs=5
  Constant2 : Constant  Value=FLT_COEF_ZERO
  Constant3 : Constant  Value=Flt_HWOverUdc_ErrCode
  Constant4 : Constant  Value=FLTLVL_FIVE
  Constant5 : Constant  Value=Flt_HWOverUdc_ActvnDetn
  Constant8 : Constant  Value=Flt_HWOverUdc_ErrDeb
  Para : Outport
  wires:
  Bus Creator/1 -> Para/1
  Constant4/1 -> Bus Creator/4  "FltLvl"
  Constant5/1 -> Bus Creator/2  "ActvnDetn"
  Constant3/1 -> Bus Creator/3  "ErrCode"
  Constant2/1 -> Bus Creator/5  "PowRecCoef"
  Constant8/1 -> Bus Creator/1  "ErrDeb"

== system FaultCheck/FaultDiag_HighTask_100us/FltDetn/OverCurrDetn/Enable ==
  Sys_SelfChkFishFlg : Inport
  Constant : Constant  Value=FLT_ON
  Constant1 : Constant  Value=FLT_ON
  Constant2 : Constant  Value=FLT_OFF
  Relational Operator : RelationalOperator  Operator===  OutDataTypeStr=boolean  RndMeth=Simplest  InputSameDT=off
  Switch : Switch  Criteria=u2 > Threshold  SaturateOnIntegerOverflow=off  InputSameDT=off
  Enable : Outport
  wires:
  Sys_SelfChkFishFlg/1 -> Relational Operator/1
  Constant/1 -> Relational Operator/2
  Relational Operator/1 -> Switch/2
  Constant1/1 -> Switch/1
  Constant2/1 -> Switch/3
  Switch/1 -> Enable/1

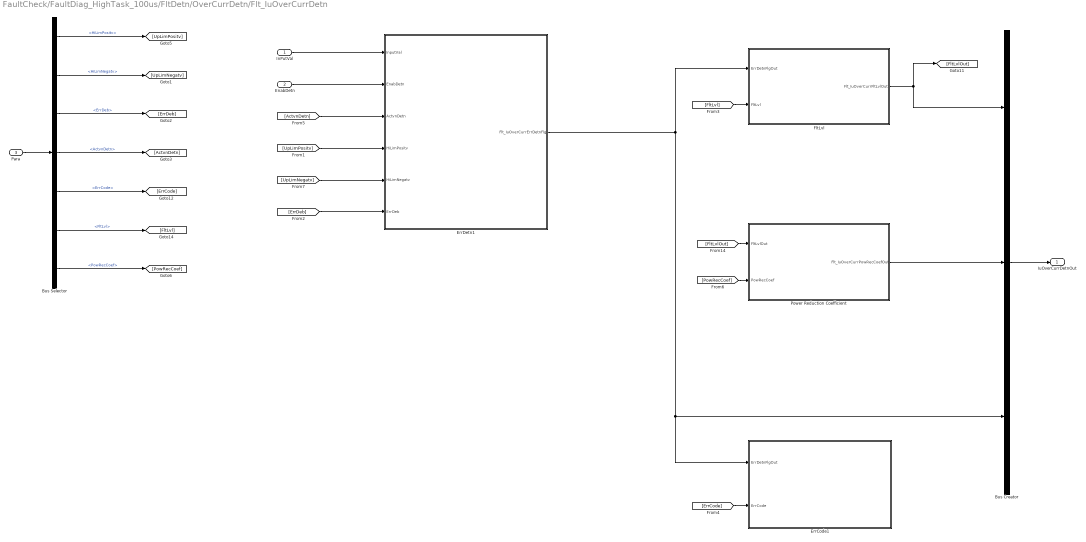
== system FaultCheck/FaultDiag_HighTask_100us/FltDetn/OverCurrDetn/Flt_IuOverCurrDetn ==
  InPutVal : Inport
  EnabDetn : Inport  Port=2
  Para : Inport  Port=3
  Bus Creator : BusCreator  Inputs=3
  Bus Selector : BusSelector  OutputSignals=HiLimPositv,HiLimNegatv,ErrDeb,ActvnDetn,ErrCode,FltLvl,PowRecCoef
  ErrCode1 : Subsystem
  ErrDetn1 : Subsystem
  FltLvl : Subsystem
  Power Reduction Coefficient : Subsystem
  IuOverCurrDetnOut : Outport
  wires:
  Para/1 -> Bus Selector/1
  Bus Selector/2 -> [UpLimNegatv]  "<HiLimNegatv>"
  Bus Selector/3 -> [ErrDeb]  "<ErrDeb>"
  ErrDetn1/1(Flt_IuOverCurrErrDetnFlg) -> Bus Creator/3, ErrCode1/1(ErrDetnFlgOut), FltLvl/1(ErrDetnFlgOut)
  FltLvl/1(Flt_IuOverCurrFltLvlOut) -> Bus Creator/1, [FltLvlOut]
  Bus Selector/5 -> [ErrCode]  "<ErrCode>"
  Bus Selector/6 -> [FltLvl]  "<FltLvl>"
  [FltLvl] -> FltLvl/2(FltLvl)
  [PowRecCoef] -> Power Reduction Coefficient/2(PowRecCoef)
  [FltLvlOut] -> Power Reduction Coefficient/1(FltLvlOut)
  [ErrDeb] -> ErrDetn1/6(ErrDeb)
  [ErrCode] -> ErrCode1/2(ErrCode)
  Power Reduction Coefficient/1(Flt_IuOverCurrPowRecCoefOut) -> Bus Creator/2
  Bus Creator/1 -> IuOverCurrDetnOut/1
  [UpLimNegatv] -> ErrDetn1/5(HiLimNegatv)
  InPutVal/1 -> ErrDetn1/1(InputVal)
  [ActvnDetn] -> ErrDetn1/3(ActvnDetn)
  EnabDetn/1 -> ErrDetn1/2(EnabDetn)
  [UpLimPositv] -> ErrDetn1/4(HiLimPositv)
  Bus Selector/1 -> [UpLimPositv]  "<HiLimPositv>"
  Bus Selector/4 -> [ActvnDetn]  "<ActvnDetn>"
  Bus Selector/7 -> [PowRecCoef]  "<PowRecCoef>"

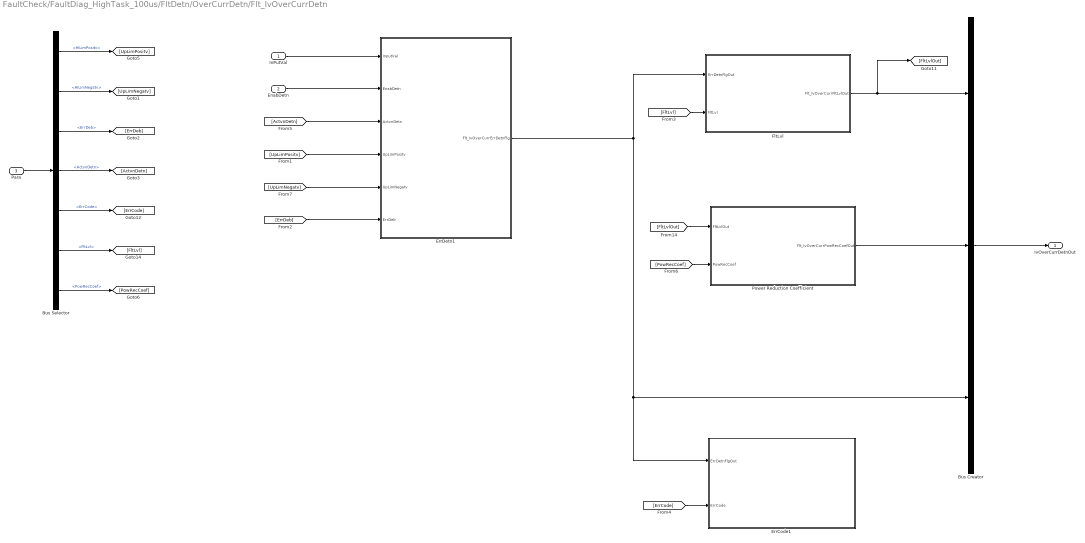
== system FaultCheck/FaultDiag_HighTask_100us/FltDetn/OverCurrDetn/Flt_IvOverCurrDetn ==
  InPutVal : Inport
  EnabDetn : Inport  Port=2
  Para : Inport  Port=3
  Bus Creator : BusCreator  Inputs=3
  Bus Selector : BusSelector  OutputSignals=HiLimPositv,HiLimNegatv,ErrDeb,ActvnDetn,ErrCode,FltLvl,PowRecCoef
  ErrCode1 : Subsystem
  ErrDetn1 : Subsystem
  FltLvl : Subsystem
  Power Reduction Coefficient : Subsystem
  IvOverCurrDetnOut : Outport
  wires:
  Bus Selector/4 -> [ActvnDetn]  "<ActvnDetn>"
  Bus Selector/1 -> [UpLimPositv]  "<HiLimPositv>"
  [UpLimPositv] -> ErrDetn1/4(UpLimPositv)
  EnabDetn/1 -> ErrDetn1/2(EnabDetn)
  [ActvnDetn] -> ErrDetn1/3(ActvnDetn)
  InPutVal/1 -> ErrDetn1/1(InputVal)
  [UpLimNegatv] -> ErrDetn1/5(UpLimNegatv)
  Bus Creator/1 -> IvOverCurrDetnOut/1
  Power Reduction Coefficient/1(Flt_IvOverCurrPowRecCoefOut) -> Bus Creator/2
  [ErrCode] -> ErrCode1/2(ErrCode)
  [ErrDeb] -> ErrDetn1/6(ErrDeb)
  [FltLvlOut] -> Power Reduction Coefficient/1(FltLvlOut)
  [PowRecCoef] -> Power Reduction Coefficient/2(PowRecCoef)
  [FltLvl] -> FltLvl/2(FltLvl)
  Bus Selector/6 -> [FltLvl]  "<FltLvl>"
  Bus Selector/5 -> [ErrCode]  "<ErrCode>"
  FltLvl/1(Flt_IvOverCurrFltLvlOut) -> [FltLvlOut], Bus Creator/1
  ErrDetn1/1(Flt_IvOverCurrErrDetnFlg) -> ErrCode1/1(ErrDetnFlgOut), Bus Creator/3, FltLvl/1(ErrDetnFlgOut)
  Bus Selector/3 -> [ErrDeb]  "<ErrDeb>"
  Bus Selector/2 -> [UpLimNegatv]  "<HiLimNegatv>"
  Para/1 -> Bus Selector/1
  Bus Selector/7 -> [PowRecCoef]  "<PowRecCoef>"

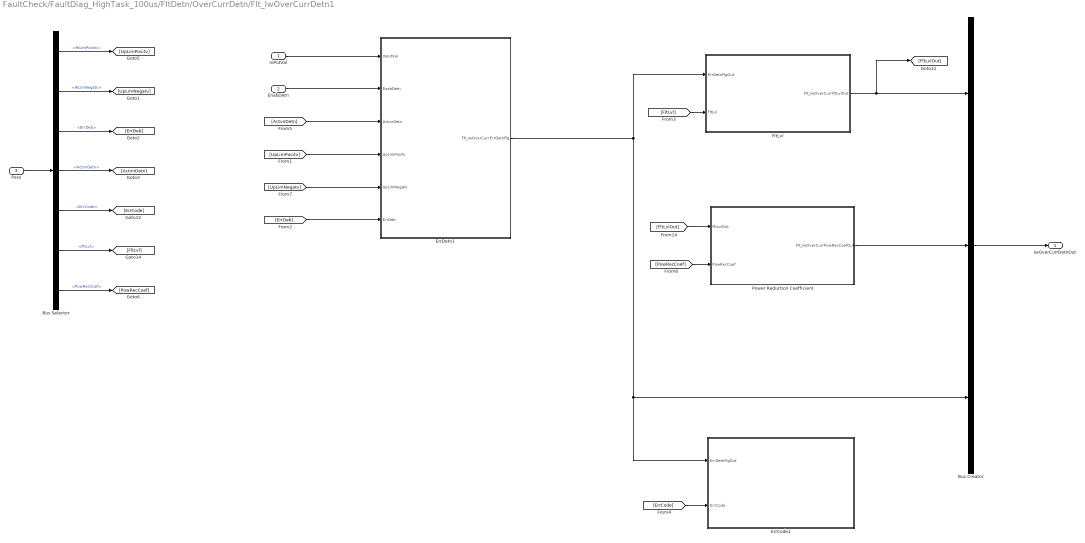
== system FaultCheck/FaultDiag_HighTask_100us/FltDetn/OverCurrDetn/Flt_IwOverCurrDetn1 ==
  InPutVal : Inport
  EnabDetn : Inport  Port=2
  Para : Inport  Port=3
  Bus Creator : BusCreator  Inputs=3
  Bus Selector : BusSelector  OutputSignals=HiLimPositv,HiLimNegatv,ErrDeb,ActvnDetn,ErrCode,FltLvl,PowRecCoef
  ErrCode1 : Subsystem
  ErrDetn1 : Subsystem
  FltLvl : Subsystem
  Power Reduction Coefficient : Subsystem
  IwOverCurrDetnOut : Outport
  wires:
  Bus Selector/4 -> [ActvnDetn]  "<ActvnDetn>"
  Bus Selector/1 -> [UpLimPositv]  "<HiLimPositv>"
  [UpLimPositv] -> ErrDetn1/4(UpLimPositv)
  EnabDetn/1 -> ErrDetn1/2(EnabDetn)
  [ActvnDetn] -> ErrDetn1/3(ActvnDetn)
  InPutVal/1 -> ErrDetn1/1(InputVal)
  [UpLimNegatv] -> ErrDetn1/5(UpLimNegatv)
  Bus Creator/1 -> IwOverCurrDetnOut/1
  Power Reduction Coefficient/1(Flt_IwOverCurrPowRecCoefOut) -> Bus Creator/2
  [ErrCode] -> ErrCode1/2(ErrCode)
  [ErrDeb] -> ErrDetn1/6(ErrDeb)
  [FltLvlOut] -> Power Reduction Coefficient/1(FltLvlOut)
  [PowRecCoef] -> Power Reduction Coefficient/2(PowRecCoef)
  [FltLvl] -> FltLvl/2(FltLvl)
  Bus Selector/6 -> [FltLvl]  "<FltLvl>"
  Bus Selector/5 -> [ErrCode]  "<ErrCode>"
  FltLvl/1(Flt_IwOverCurrFltLvlOut) -> [FltLvlOut], Bus Creator/1
  ErrDetn1/1(Flt_IwOverCurrErrDetnFlg) -> ErrCode1/1(ErrDetnFlgOut), Bus Creator/3, FltLvl/1(ErrDetnFlgOut)
  Bus Selector/3 -> [ErrDeb]  "<ErrDeb>"
  Bus Selector/2 -> [UpLimNegatv]  "<HiLimNegatv>"
  Para/1 -> Bus Selector/1
  Bus Selector/7 -> [PowRecCoef]  "<PowRecCoef>"

== system FaultCheck/FaultDiag_HighTask_100us/FltDetn/OverCurrDetn/Parameter ==
  Bus Creator : BusCreator  Inputs=7
  Constant1 : Constant  Value=Flt_IuOverCurr_HiLimNegatv
  Constant11 : Constant  Value=Flt_IuOverCurr_ErrCode
  Constant13 : Constant  Value=FLTLVL_FOUR
  Constant2 : Constant  Value=FLT_COEF_ZERO
  Constant6 : Constant  Value=Flt_IuOverCurr_ActvErrDetn
  Constant7 : Constant  Value=Flt_IuOverCurr_HiLimPositv
  Constant8 : Constant  Value=Flt_IuOverCurr_ErrDeb
  Para : Outport
  wires:
  Constant7/1 -> Bus Creator/1  "HiLimPositv"
  Constant13/1 -> Bus Creator/6  "FltLvl"
  Constant11/1 -> Bus Creator/5  "ErrCode"
  Bus Creator/1 -> Para/1
  Constant1/1 -> Bus Creator/2  "HiLimNegatv"
  Constant8/1 -> Bus Creator/3  "ErrDeb"
  Constant6/1 -> Bus Creator/4  "ActvnDetn"
  Constant2/1 -> Bus Creator/7  "PowRecCoef"

== system FaultCheck/FaultDiag_HighTask_100us/FltDetn/OverCurrDetn/Parameter1 ==
  Bus Creator : BusCreator  Inputs=7
  Constant1 : Constant  Value=Flt_IvOverCurr_HiLimNegatv
  Constant11 : Constant  Value=Flt_IvOverCurr_ErrCode
  Constant13 : Constant  Value=FLTLVL_FOUR
  Constant2 : Constant  Value=FLT_COEF_ZERO
  Constant6 : Constant  Value=Flt_IvOverCurr_ActvErrDetn
  Constant7 : Constant  Value=Flt_IvOverCurr_HiLimPositv
  Constant8 : Constant  Value=Flt_IvOverCurr_ErrDeb
  Para : Outport
  wires:
  Constant6/1 -> Bus Creator/4  "ActvnDetn"
  Constant8/1 -> Bus Creator/3  "ErrDeb"
  Constant1/1 -> Bus Creator/2  "HiLimNegatv"
  Bus Creator/1 -> Para/1
  Constant11/1 -> Bus Creator/5  "ErrCode"
  Constant13/1 -> Bus Creator/6  "FltLvl"
  Constant7/1 -> Bus Creator/1  "HiLimPositv"
  Constant2/1 -> Bus Creator/7  "PowRecCoef"

== system FaultCheck/FaultDiag_HighTask_100us/FltDetn/OverCurrDetn/Parameter2 ==
  Bus Creator : BusCreator  Inputs=7
  Constant1 : Constant  Value=Flt_IwOverCurr_HiLimNegatv
  Constant11 : Constant  Value=Flt_IwOverCurr_ErrCode
  Constant13 : Constant  Value=FLTLVL_FOUR
  Constant2 : Constant  Value=FLT_COEF_ZERO
  Constant6 : Constant  Value=Flt_IwOverCurr_ActvErrDetn
  Constant7 : Constant  Value=Flt_IwOverCurr_HiLimPositv
  Constant8 : Constant  Value=Flt_IwOverCurr_ErrDeb
  Para : Outport
  wires:
  Constant6/1 -> Bus Creator/4  "ActvnDetn"
  Constant8/1 -> Bus Creator/3  "ErrDeb"
  Constant1/1 -> Bus Creator/2  "HiLimNegatv"
  Bus Creator/1 -> Para/1
  Constant11/1 -> Bus Creator/5  "ErrCode"
  Constant13/1 -> Bus Creator/6  "FltLvl"
  Constant7/1 -> Bus Creator/1  "HiLimPositv"
  Constant2/1 -> Bus Creator/7  "PowRecCoef"

== system FaultCheck/FaultDiag_HighTask_100us/FltDetn/RecUDetn/Enable ==
  Sys_SelfChkFishFlg : Inport
  Constant : Constant  Value=FLT_ON
  Constant1 : Constant  Value=FLT_ON
  Constant2 : Constant  Value=FLT_OFF
  Relational Operator : RelationalOperator  Operator===  OutDataTypeStr=boolean  RndMeth=Simplest  InputSameDT=off
  Switch : Switch  Criteria=u2 > Threshold  SaturateOnIntegerOverflow=off  InputSameDT=off
  Enable : Outport
  wires:
  Switch/1 -> Enable/1
  Constant2/1 -> Switch/3
  Constant1/1 -> Switch/1
  Relational Operator/1 -> Switch/2
  Constant/1 -> Relational Operator/2
  Sys_SelfChkFishFlg/1 -> Relational Operator/1

== system FaultCheck/FaultDiag_HighTask_100us/FltDetn/RecUDetn/Parameter ==
  Bus Creator : BusCreator  Inputs=5
  Constant2 : Constant  Value=FLT_COEF_ZERO
  Constant3 : Constant  Value=Flt_RecU_ErrCode
  Constant4 : Constant  Value=FLTLVL_FIVE
  Constant5 : Constant  Value=Flt_RecU_ActvnErrDetn
  Constant8 : Constant  Value=Flt_RecU_ErrDeb
  Para : Outport
  wires:
  Bus Creator/1 -> Para/1
  Constant4/1 -> Bus Creator/4  "FltLvl"
  Constant5/1 -> Bus Creator/2  "ActvnDetn"
  Constant3/1 -> Bus Creator/3  "ErrCode"
  Constant2/1 -> Bus Creator/5  "PowRecCoef"
  Constant8/1 -> Bus Creator/1  "ErrDeb"

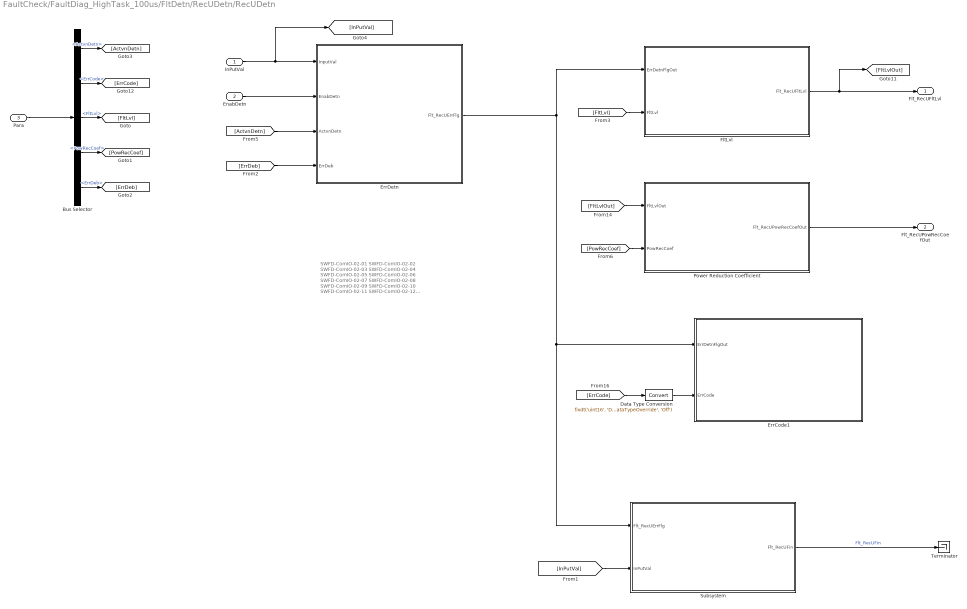
== system FaultCheck/FaultDiag_HighTask_100us/FltDetn/RecUDetn/RecUDetn ==
  note: SWFD-ComIO-02-01
      |
      | SWFD-ComIO-02-02
      |
      | SWFD-ComIO-02-03
      |
      | SWFD-ComIO-02-04
      |
      | SWFD-ComIO-02-05
      |
      | SWFD-ComIO-02-06
      |
      | SWFD-ComIO-02-07
      |
      | SWFD-ComIO-02-08
      |
      | SWFD-ComIO-02-09
      |
      | SWFD-ComIO-02-10
      |
      | SWFD-ComIO-02-11
      |
      | SWFD-ComIO-02-12
      |
      | SWFD-ResVolt-11-01
      |
      | SWFD-ResVolt-11-02
      |
      | SWFD-ResVolt-11-03
  InPutVal : Inport
  EnabDetn : Inport  Port=2
  Para : Inport  Port=3
  Bus Selector : BusSelector  OutputSignals=ActvnDetn,ErrCode,FltLvl,PowRecCoef,ErrDeb
  Data Type Conversion : DataTypeConversion  OutDataTypeStr=fixdt('uint16', 'DataTypeOverride', 'Off')  SaturateOnIntegerOverflow=off  RndMeth=Floor
  ErrCode1 : Subsystem
  ErrDetn : Subsystem
  FltLvl : Subsystem
  Power Reduction Coefficient : Subsystem
  Subsystem : Subsystem
  Terminator : Terminator
  Flt_RecUFltLvl : Outport
  Flt_RecUPowRecCoefOut : Outport  Port=2
  wires:
  ErrDetn/1(Flt_RecUErrFlg) -> ErrCode1/1(ErrDetnFlgOut), Subsystem/1(Flt_RecUErrFlg), FltLvl/1(ErrDetnFlgOut)
  Subsystem/1(Flt_RecUFin) -> Terminator/1  "Flt_RecUFin"
  [InPutVal] -> Subsystem/2(InPutVal)
  Bus Selector/5 -> [ErrDeb]  "<ErrDeb>"
  Power Reduction Coefficient/1(Flt_RecUPowRecCoefOut) -> Flt_RecUPowRecCoefOut/1
  [PowRecCoef] -> Power Reduction Coefficient/2(PowRecCoef)
  [FltLvlOut] -> Power Reduction Coefficient/1(FltLvlOut)
  [FltLvl] -> FltLvl/2(FltLvl)
  FltLvl/1(Flt_RecUFltLvl) -> Flt_RecUFltLvl/1, [FltLvlOut]
  [ErrCode] -> Data Type Conversion/1
  Para/1 -> Bus Selector/1
  Bus Selector/1 -> [ActvnDetn]  "<ActvnDetn>"
  Bus Selector/2 -> [ErrCode]  "<ErrCode>"
  Bus Selector/3 -> [FltLvl]  "<FltLvl>"
  Bus Selector/4 -> [PowRecCoef]  "<PowRecCoef>"
  [ErrDeb] -> ErrDetn/4(ErrDeb)
  EnabDetn/1 -> ErrDetn/2(EnabDetn)
  [ActvnDetn] -> ErrDetn/3(ActvnDetn)
  InPutVal/1 -> ErrDetn/1(InputVal), [InPutVal]
  Data Type Conversion/1 -> ErrCode1/2(ErrCode)

== system FaultCheck/FaultDiag_HighTask_100us/FltDetn/ResErrFlgDetn/Enable ==
  Sys_SelfChkFishFlg : Inport
  Constant : Constant  Value=FLT_ON
  Constant1 : Constant  Value=FLT_ON
  Constant2 : Constant  Value=FLT_OFF
  Relational Operator : RelationalOperator  Operator===  OutDataTypeStr=boolean  RndMeth=Simplest  InputSameDT=off
  Switch : Switch  Criteria=u2 > Threshold  SaturateOnIntegerOverflow=off  InputSameDT=off
  Enable : Outport
  wires:
  Sys_SelfChkFishFlg/1 -> Relational Operator/1
  Constant/1 -> Relational Operator/2
  Relational Operator/1 -> Switch/2
  Constant1/1 -> Switch/1
  Constant2/1 -> Switch/3
  Switch/1 -> Enable/1

== system FaultCheck/FaultDiag_HighTask_100us/FltDetn/ResErrFlgDetn/Parameter ==
  Bus Creator : BusCreator  Inputs=4
  Constant2 : Constant  Value=FLT_COEF_ZERO
  Constant3 : Constant  Value=Flt_ResErr_ErrCode
  Constant4 : Constant  Value=FLTLVL_FIVE
  Constant5 : Constant  Value=Flt_ResErr_ActvnDetn
  Para : Outport
  wires:
  Bus Creator/1 -> Para/1
  Constant4/1 -> Bus Creator/3  "FltLvl"
  Constant5/1 -> Bus Creator/1  "ActvnDetn"
  Constant3/1 -> Bus Creator/2  "ErrCode"
  Constant2/1 -> Bus Creator/4  "PowRecCoef"

== system FaultCheck/FaultDiag_HighTask_100us/FltDetn/ResErrFlgDetn/ResErrDetn ==
  InPutVal1 : Inport
  EnabDetn : Inport  Port=2
  Para : Inport  Port=3
  Bus Selector : BusSelector  OutputSignals=ActvnDetn,ErrCode,FltLvl,PowRecCoef
  ErrCode : Subsystem
  ErrDetn : Subsystem
  FltLvl : Subsystem
  Power Reduction Coefficient : Subsystem
  Flt_ResErrFltLvl : Outport
  Flt_ResErrPowRecCoefOut : Outport  Port=2
  wires:
  Power Reduction Coefficient/1(Flt_ResErrPowRecCoefOut) -> Flt_ResErrPowRecCoefOut/1
  [PowRecCoef] -> Power Reduction Coefficient/2(PowRecCoef)
  [FltLvlOut] -> Power Reduction Coefficient/1(FltLvlOut)
  [FltLvl] -> FltLvl/2(FltLvl)
  FltLvl/1(Flt_ResErrFltLvl) -> Flt_ResErrFltLvl/1, [FltLvlOut]
  [ErrCode] -> ErrCode/2(ErrCode)
  Para/1 -> Bus Selector/1
  Bus Selector/1 -> [ActvnDetn]  "<ActvnDetn>"
  Bus Selector/2 -> [ErrCode]  "<ErrCode>"
  Bus Selector/3 -> [FltLvl]  "<FltLvl>"
  Bus Selector/4 -> [PowRecCoef]  "<PowRecCoef>"
  EnabDetn/1 -> ErrDetn/2(EnabDetn)
  [ActvnDetn] -> ErrDetn/3(ActvnDetn)
  InPutVal1/1 -> ErrDetn/1(InputVal)
  ErrDetn/1(Flt_ResErrErrFlg) -> ErrCode/1(ErrDetnFlgOut), FltLvl/1(ErrDetnFlgOut)

== system FaultCheck/FaultDiag_HighTask_100us/FltDetn/ResolveSensorDetn/Enable ==
  Sys_SelfChkFishFlg : Inport
  Constant : Constant  Value=FLT_ON
  Constant1 : Constant  Value=FLT_ON
  Constant2 : Constant  Value=FLT_OFF
  Relational Operator : RelationalOperator  Operator===  OutDataTypeStr=boolean  RndMeth=Simplest  InputSameDT=off
  Switch : Switch  Criteria=u2 > Threshold  SaturateOnIntegerOverflow=off  InputSameDT=off
  Enable : Outport
  wires:
  Switch/1 -> Enable/1
  Constant2/1 -> Switch/3
  Constant1/1 -> Switch/1
  Relational Operator/1 -> Switch/2
  Constant/1 -> Relational Operator/2
  Sys_SelfChkFishFlg/1 -> Relational Operator/1

== system FaultCheck/FaultDiag_HighTask_100us/FltDetn/ResolveSensorDetn/Flt_ResolveSensorDetn ==
  InPutVal1 : Inport
  EnabDetn : Inport  Port=2
  Para : Inport  Port=3
  Bus Selector : BusSelector  OutputSignals=ActvnDetn,ErrCode,FltLvl,PowRecCoef,ErrDeb
  Data Type Conversion : DataTypeConversion  OutDataTypeStr=fixdt('uint16', 'DataTypeOverride', 'Off')  SaturateOnIntegerOverflow=off  RndMeth=Floor
  ErrCode : Subsystem
  ErrDetn : Subsystem
  FltLvl : Subsystem
  Power Reduction Coefficient : Subsystem
  Flt_ResolveSensorFltLvl : Outport
  Flt_ResolveSensorPowRecCoefOut : Outport  Port=2
  wires:
  Bus Selector/5 -> [ErrDeb]  "<ErrDeb>"
  ErrDetn/1(Flt_ResolveSensorErrFlg) -> FltLvl/1(ErrDetnFlgOut), ErrCode/1(ErrDetnFlgOut)
  InPutVal1/1 -> ErrDetn/1(InputVal)
  [ActvnDetn] -> ErrDetn/3(ActvnDetn)
  EnabDetn/1 -> ErrDetn/2(EnabDetn)
  [ErrDeb] -> ErrDetn/4(ErrDeb)
  Bus Selector/4 -> [PowRecCoef]  "<PowRecCoef>"
  Bus Selector/3 -> [FltLvl]  "<FltLvl>"
  Bus Selector/2 -> [ErrCode]  "<ErrCode>"
  Bus Selector/1 -> [ActvnDetn]  "<ActvnDetn>"
  Para/1 -> Bus Selector/1
  [ErrCode] -> Data Type Conversion/1
  FltLvl/1(Flt_ResolveSensorFltLvl) -> [FltLvlOut], Flt_ResolveSensorFltLvl/1
  [FltLvl] -> FltLvl/2(FltLvl)
  [FltLvlOut] -> Power Reduction Coefficient/1(FltLvlOut)
  [PowRecCoef] -> Power Reduction Coefficient/2(PowRecCoef)
  Power Reduction Coefficient/1(Flt_ResolveSensorPowRecCoefOut) -> Flt_ResolveSensorPowRecCoefOut/1
  Data Type Conversion/1 -> ErrCode/2(ErrCode)

== system FaultCheck/FaultDiag_HighTask_100us/FltDetn/ResolveSensorDetn/Parameter ==
  Bus Creator : BusCreator  Inputs=5
  Constant2 : Constant  Value=FLT_COEF_ZERO
  Constant3 : Constant  Value=Flt_ResolveSensor_ErrCode
  Constant4 : Constant  Value=FLTLVL_FIVE
  Constant5 : Constant  Value=Flt_ResolveSensor_ActvnDetn
  Constant8 : Constant  Value=Flt_ResolveSensor_ErrDeb
  Para : Outport
  wires:
  Constant8/1 -> Bus Creator/1  "ErrDeb"
  Constant2/1 -> Bus Creator/5  "PowRecCoef"
  Constant3/1 -> Bus Creator/3  "ErrCode"
  Constant5/1 -> Bus Creator/2  "ActvnDetn"
  Constant4/1 -> Bus Creator/4  "FltLvl"
  Bus Creator/1 -> Para/1

== system FaultCheck/FaultDiag_HighTask_100us/FltDetn/UdcDetn/Enable ==
  Sys_EMWorkMode : Inport
  Sys_SelfChkFishFlg : Inport  Port=2
  AND : Logic  AllPortsSameDT=off  OutDataTypeStr=boolean
  Compare To Constant : simulink/Logic and Bit Operations/Compare To Constant  relop===  const=FLT_ON  OutDataTypeStr=boolean
  Compare To Constant2 : simulink/Logic and Bit Operations/Compare To Constant  relop===  const=EMWorkMode_enum_tqmode  OutDataTypeStr=boolean
  Compare To Constant3 : simulink/Logic and Bit Operations/Compare To Constant  relop===  const=EMWorkMode_enum_spdmode  OutDataTypeStr=boolean
  Compare To Constant4 : simulink/Logic and Bit Operations/Compare To Constant  relop===  const=EMWorkMode_enum_debug  OutDataTypeStr=boolean
  Constant1 : Constant  Value=FLT_ON
  Constant2 : Constant  Value=FLT_OFF
  Logical Operator3 : Logic  Operator=OR  Inputs=3  AllPortsSameDT=off  OutDataTypeStr=boolean
  Switch : Switch  Criteria=u2 ~= 0  SaturateOnIntegerOverflow=off  InputSameDT=off
  Enable : Outport
  Enable1 : Outport  Port=2
  wires:
  Compare To Constant4/1 -> Logical Operator3/3
  Compare To Constant3/1 -> Logical Operator3/2
  Compare To Constant2/1 -> Logical Operator3/1
  Sys_EMWorkMode/1 -> Compare To Constant2/1, Compare To Constant3/1, Compare To Constant4/1
  AND/1 -> Switch/2
  Compare To Constant/1 -> AND/2, Enable1/1
  Logical Operator3/1 -> AND/1
  Sys_SelfChkFishFlg/1 -> Compare To Constant/1
  Switch/1 -> Enable/1
  Constant2/1 -> Switch/3
  Constant1/1 -> Switch/1

== system FaultCheck/FaultDiag_HighTask_100us/FltDetn/UdcDetn/Parameter ==
  IPC_UdcRaw_mV : Inport
  Bus Creator : BusCreator  Inputs=8
  Constant11 : Constant  Value=Flt_UdcUnderLim1_ErrCode
  Constant13 : Constant  Value=FLTLVL_TWO
  Constant2 : Constant  Value=Flt_UdcUnderLim1_RecLim1
  Constant3 : Constant  Value=Flt_UdcUnderLim1_RecDeb
  Constant6 : Constant  Value=Flt_UdcUnderLim1_ActvErrDetn
  Constant7 : Constant  Value=Flt_UdcUnderLim1_LoLim1
  Constant8 : Constant  Value=Flt_UdcUnderLim1_ErrDeb
  Flt_UdcUnderLim1_PowRecCoef : Lookup_n-D  NumberOfTableDimensions=1  BreakpointsForDimension1=Flt_UdcRawLo1_V  BreakpointsForDimension1DataTypeStr=Inherit: Inherit from 'Breakpoint data'  Table=Flt_UdcUnderLim1_PowRecCoef  TableDataTypeStr=Inherit: Inherit from 'Table data'  ExtrapMethod=Clip  UseLastTableValue=on  InternalRulePriority=Speed  OutDataTypeStr=Inherit: Inherit from 'Table data'  RndMeth=Simplest  MaximumIndicesForEachDimension=[1 5]
  Para : Outport
  wires:
  IPC_UdcRaw_mV/1 -> Flt_UdcUnderLim1_PowRecCoef/1
  Bus Creator/1 -> Para/1
  Constant11/1 -> Bus Creator/6  "ErrCode"
  Constant13/1 -> Bus Creator/7  "FltLvl"
  Flt_UdcUnderLim1_PowRecCoef/1 -> Bus Creator/8  "PowRecCoef"
  Constant7/1 -> Bus Creator/1  "LoLim1"
  Constant8/1 -> Bus Creator/2  "ErrDeb"
  Constant6/1 -> Bus Creator/3  "ActvnDetn"
  Constant3/1 -> Bus Creator/5  "RecDeb"
  Constant2/1 -> Bus Creator/4  "RecLim1"

== system FaultCheck/FaultDiag_HighTask_100us/FltDetn/UdcDetn/Parameter1 ==
  Bus Creator : BusCreator  Inputs=8
  Constant1 : Constant  Value=FLT_COEF_ZERO
  Constant11 : Constant  Value=Flt_UdcUnderLim2_ErrCode
  Constant13 : Constant  Value=FLTLVL_THREE
  Constant2 : Constant  Value=Flt_UdcUnderLim2_RecLim2
  Constant3 : Constant  Value=Flt_UdcUnderLim2_RecDeb
  Constant6 : Constant  Value=Flt_UdcUnderLim2_ActvErrDetn
  Constant7 : Constant  Value=Flt_UdcUnderLim2_LoLim2
  Constant8 : Constant  Value=Flt_UdcUnderLim2_ErrDeb
  Para : Outport
  wires:
  Constant2/1 -> Bus Creator/4  "RecLim2"
  Constant3/1 -> Bus Creator/5  "RecDeb"
  Constant6/1 -> Bus Creator/3  "ActvnDetn"
  Constant8/1 -> Bus Creator/2  "ErrDeb"
  Constant7/1 -> Bus Creator/1  "LoLim2"
  Constant1/1 -> Bus Creator/8  "PowRecCoef"
  Constant13/1 -> Bus Creator/7  "FltLvl"
  Constant11/1 -> Bus Creator/6  "ErrCode"
  Bus Creator/1 -> Para/1
